simulink subsystem "PID_Vel"  (R2026a)
settings: Solver=VariableStepAuto
values from neighbouring files (symbols this model uses):
  Kd = 1    [coeficientes.m]
  Ki = 1    [coeficientes.m]
  Kp = 1    [coeficientes.m]
settings Model: Creator=admin  LastModifiedBy=admin

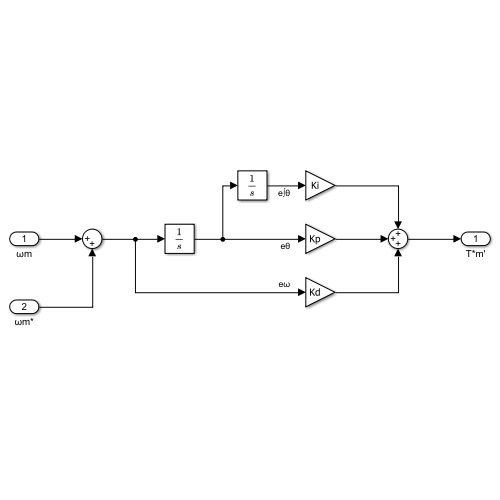
[thumbnail: Simulink's stored preview of the top-level diagram]
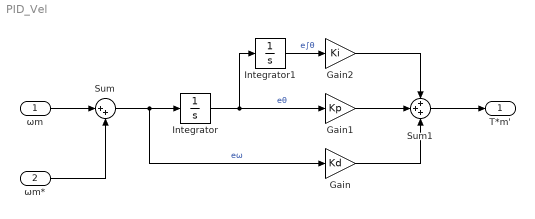
== system PID_Vel ==
  ωm : Inport  Unit=rad/s
  ωm* : Inport  Port=2  Unit=rad/s
  Gain : Gain  Gain=Kd
  Gain1 : Gain  Gain=Kp
  Gain2 : Gain  Gain=Ki
  Integrator : Integrator
  Integrator1 : Integrator
  Sum : Sum  Inputs=|++
  Sum1 : Sum  Inputs=+++
  T*m' : Outport
  wires:
  Gain1/1 -> Sum1/2
  Gain/1 -> Sum1/3
  Integrator/1 -> Integrator1/1, Gain1/1  "eθ"
  ωm/1 -> Sum/1
  Sum1/1 -> T*m'/1
  ωm*/1 -> Sum/2
  Integrator1/1 -> Gain2/1  "e∫θ"
  Sum/1 -> Gain/1, Integrator/1  "eω"
  Gain2/1 -> Sum1/1
